simulink model "IHC_Lowpass_Filter"  (R2019b)
settings: Solver=VariableStepAuto  StartTime=0.0  StopTime=testtime  RelTol=1e-3
InitFcn:
  | IHC_Lowpass_Test_Parameters
StopFcn:
  | Verify_IHC_Lowpass_Filter
values from neighbouring files (symbols this model uses):
  c1LPihc = ( C - TWOPI*Fcihc ) / ( C + TWOPI*Fcihc )    (= 0.671752219322)    [IHC_Lowpass_Test_Parameters.m]
  c2LPihc = TWOPI*Fcihc / (TWOPI*Fcihc + C)    (= 0.164123890339)    [IHC_Lowpass_Test_Parameters.m]
  Fs = 48e3    (= 48000)    [IHC_Lowpass_Test_Parameters.m]
  gainihc = 1.0    (= 1)    [IHC_Lowpass_Test_Parameters.m]
undefined symbols (not defined in the file or in its folder): dfilt
libraries: dsparch4 x4, dspsrcs4 x2
settings Model: Creator=mblun  LastModifiedBy=cb50701
settings SFSimCC: CustomCodeUndefinedFunction=UseInterfaceOnly

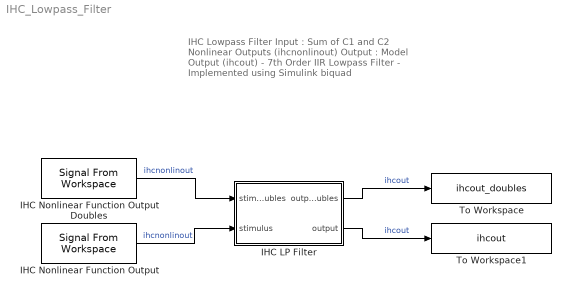
== system IHC_Lowpass_Filter ==
  note: IHC Lowpass Filter
      |
      | Input : Sum of C1 and C2 Nonlinear Outputs (ihcnonlinout)
      |
      | Output : Model Output (ihcout)
      |
      | - 7th Order IIR Lowpass Filter
      |
      | - Implemented using Simulink biquad
  IHC LP Filter : Subsystem
  IHC Nonlinear Function Output : dspsrcs4/Signal From Workspace  X=RxSignal  Ts=1/Fs  nsamps=1  OutputAfterFinalValue=Setting to zero  ignoreOrWarnInputAndFrameLengths=off  OutputFrames=off
  IHC Nonlinear Function Output Doubles : dspsrcs4/Signal From Workspace  X=RxSignal_doubles  Ts=1/Fs  nsamps=1  OutputAfterFinalValue=Setting to zero  ignoreOrWarnInputAndFrameLengths=off  OutputFrames=off
  To Workspace : ToWorkspace  VariableName=ihcout_doubles  SampleTime=-1
      settings: Save2DSignal=2-D array (concatenate along first dimension)
  To Workspace1 : ToWorkspace  VariableName=ihcout  SampleTime=-1
      settings: Save2DSignal=2-D array (concatenate along first dimension)
  wires:
  IHC Nonlinear Function Output Doubles/1 -> IHC LP Filter/1(stimulus_doubles)  "ihcnonlinout"
  IHC LP Filter/2(output) -> To Workspace1/1  "ihcout"
  IHC Nonlinear Function Output/1 -> IHC LP Filter/2(stimulus)  "ihcnonlinout"
  IHC LP Filter/1(output_doubles) -> To Workspace/1  "ihcout"

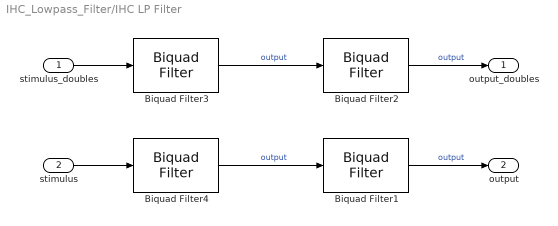
== system IHC_Lowpass_Filter/IHC LP Filter ==
  stimulus_doubles : Inport
  stimulus : Inport  Port=2
  Biquad Filter1 : dsparch4/Biquad Filter  FilterSource=Dialog parameters  CoeffSource=Specify via dialog  FilterObject=dfilt.df2tsos([1 0.3 0.4],[1 0.1 0.2])  IIRFiltStruct=Direct form II transposed  BiQuadCoeffs=[c2LPihc c2LPihc 0 1 -c1LPihc 0; c2LPihc c2LPihc 0 1 -c1LPihc 0; c2LPihc c2LPihc 0 1 -c1LPihc 0]  ScaleValues=1  IC=0  ICnum=0  ICden=0  a0Flag=Warning  optimizeScaleValues=on  ScaleValueMode=Specify via input port (g)  roundingMode=Floor  overflowMode=on  scaleValueFracLength=14  denProdOutputFracLength=30  denAccumFracLength=30  secondMemoryFracLength=15
      settings: SourceProductName=DSP System Toolbox
  Biquad Filter2 : dsparch4/Biquad Filter  FilterSource=Dialog parameters  CoeffSource=Specify via dialog  FilterObject=dfilt.df2tsos([1 0.3 0.4],[1 0.1 0.2])  IIRFiltStruct=Direct form II transposed  BiQuadCoeffs=[c2LPihc c2LPihc 0 1 -c1LPihc 0; c2LPihc c2LPihc 0 1 -c1LPihc 0; c2LPihc c2LPihc 0 1 -c1LPihc 0]  ScaleValues=1  IC=0  ICnum=0  ICden=0  a0Flag=Warning  optimizeScaleValues=on  ScaleValueMode=Specify via input port (g)  roundingMode=Floor  overflowMode=on  scaleValueFracLength=14  denProdOutputFracLength=30  denAccumFracLength=30  secondMemoryFracLength=15
      settings: SourceProductName=DSP System Toolbox
  Biquad Filter3 : dsparch4/Biquad Filter  FilterSource=Dialog parameters  CoeffSource=Specify via dialog  FilterObject=dfilt.df2tsos([1 0.3 0.4],[1 0.1 0.2])  IIRFiltStruct=Direct form II transposed  BiQuadCoeffs=[gainihc*c2LPihc gainihc*c2LPihc 0 1 -c1LPihc 0; c2LPihc c2LPihc 0 1 -c1LPihc 0; c2LPihc c2LPihc 0 1 -c1LPihc 0;c2LPihc c2LPihc 0 1 -c1LPihc 0]  ScaleValues=1  IC=0  ICnum=0  ICden=0  a0Flag=Warning  optimizeScaleValues=on  ScaleValueMode=Specify via input port (g)  roundingMode=Floor  overflowMode=on  scaleValueFracLength=14  denProdOutputFracLength=30  denAccumFracLength=30  secondMemoryFracLength=15
      settings: SourceProductName=DSP System Toolbox
  Biquad Filter4 : dsparch4/Biquad Filter  FilterSource=Dialog parameters  CoeffSource=Specify via dialog  FilterObject=dfilt.df2tsos([1 0.3 0.4],[1 0.1 0.2])  IIRFiltStruct=Direct form II transposed  BiQuadCoeffs=[gainihc*c2LPihc gainihc*c2LPihc 0 1 -c1LPihc 0; c2LPihc c2LPihc 0 1 -c1LPihc 0; c2LPihc c2LPihc 0 1 -c1LPihc 0;c2LPihc c2LPihc 0 1 -c1LPihc 0]  ScaleValues=1  IC=0  ICnum=0  ICden=0  a0Flag=Warning  optimizeScaleValues=on  ScaleValueMode=Specify via input port (g)  roundingMode=Floor  overflowMode=on  scaleValueFracLength=14  denProdOutputFracLength=30  denAccumFracLength=30  secondMemoryFracLength=15
      settings: SourceProductName=DSP System Toolbox
  output_doubles : Outport  VectorParamsAs1DForOutWhenUnconnected=off
  output : Outport  Port=2  VectorParamsAs1DForOutWhenUnconnected=off
  wires:
  stimulus/1 -> Biquad Filter4/1
  Biquad Filter4/1 -> Biquad Filter1/1  "output"
  Biquad Filter1/1 -> output/1  "output"
  stimulus_doubles/1 -> Biquad Filter3/1
  Biquad Filter3/1 -> Biquad Filter2/1  "output"
  Biquad Filter2/1 -> output_doubles/1  "output"
